simulink library "waveFlow_ul"  (R2018b)
settings: Solver=VariableStepAuto  StartTime=0.0  StopTime=10.0  RelTol=1e-3
undefined symbols (not defined in the file): e, initializeBussesFromBlock
settings Model: Creator=mcobb  LastModifiedBy=mcobb

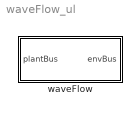
== system waveFlow_ul ==
  waveFlow : Subsystem  LoadFcn=initializeBussesFromBlock(gcb)  InitFcn=initializeBussesFromBlock(gcb)  StartFcn=initializeBussesFromBlock(gcb)  mask{e=e}
      mask prompts: e "Wave Flow Object"

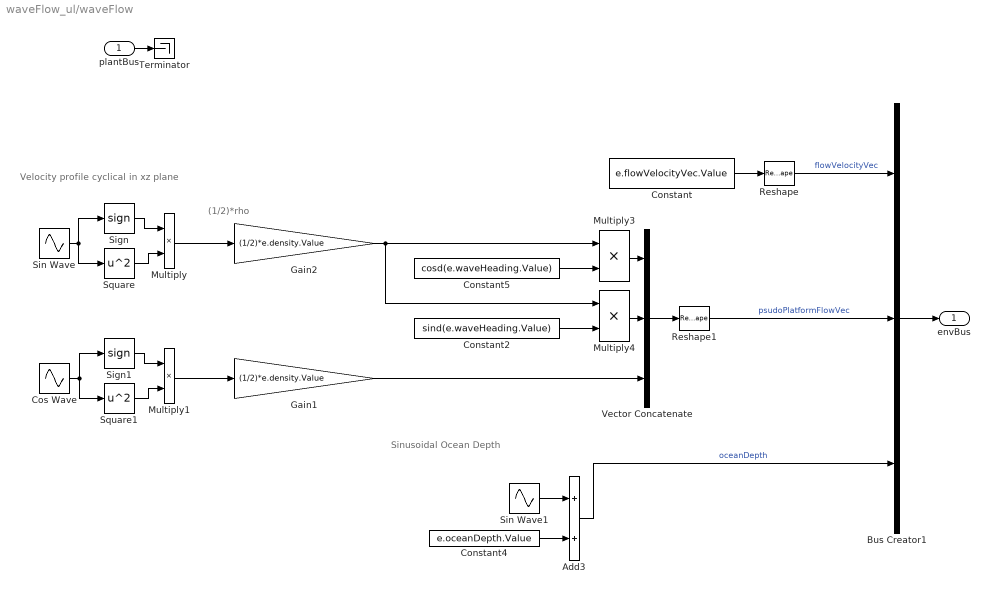
== system waveFlow_ul/waveFlow ==
  note: (1/2)*rho
  note: Velocity profile cyclical
      | in xz plane
  note: Sinusoidal Ocean Depth
  plantBus : Inport  OutDataTypeStr=Bus: plantBus
  Add3 : Sum
  Bus Creator1 : BusCreator  Inputs=3  OutDataTypeStr=Bus:envBus
  Constant : Constant  Value=e.flowVelocityVec.Value
  Constant2 : Constant  Value=sind(e.waveHeading.Value)
  Constant4 : Constant  Value=e.oceanDepth.Value
  Constant5 : Constant  Value=cosd(e.waveHeading.Value)
  Cos Wave : Sin  Amplitude=e.pltfrmAppFlwMag.Value  Frequency=2*pi/e.wavePeriod.Value  Phase=pi/2  SampleTime=0
  Gain1 : Gain  Gain=(1/2)*e.density.Value
  Gain2 : Gain  Gain=(1/2)*e.density.Value
  Multiply{,1,3..4} (4 alike) : Product
  Reshape : Reshape  OutputDimensionality=Column vector (2-D)
  Reshape1 : Reshape  OutputDimensionality=Column vector (2-D)
  Sign : Signum
  Sign1 : Signum
  Sin Wave : Sin  Amplitude=e.pltfrmAppFlwMag.Value  Frequency=2*pi/e.wavePeriod.Value  SampleTime=0
  Sin Wave1 : Sin  Amplitude=e.waveAmplitude.Value  Frequency=2*pi/e.wavePeriod.Value  SampleTime=0
  Square : Math  Operator=square  SaturateOnIntegerOverflow=on
  Square1 : Math  Operator=square  SaturateOnIntegerOverflow=on
  Terminator : Terminator
  Vector Concatenate : Concatenate  NumInputs=3
  envBus : Outport  OutDataTypeStr=Bus: envBus
  wires:
  Bus Creator1/1 -> envBus/1
  Constant/1 -> Reshape/1
  Reshape/1 -> Bus Creator1/1  "flowVelocityVec"
  Reshape1/1 -> Bus Creator1/2  "psudoPlatformFlowVec"
  Vector Concatenate/1 -> Reshape1/1
  Gain1/1 -> Vector Concatenate/3
  Gain2/1 -> Multiply3/1, Multiply4/1
  Sin Wave/1 -> Square/1, Sign/1
  Multiply/1 -> Gain2/1
  Square/1 -> Multiply/2
  Sign/1 -> Multiply/1
  Sign1/1 -> Multiply1/1
  Square1/1 -> Multiply1/2
  Multiply1/1 -> Gain1/1
  Cos Wave/1 -> Sign1/1, Square1/1
  Sin Wave1/1 -> Add3/1
  Add3/1 -> Bus Creator1/3  "oceanDepth"
  Constant4/1 -> Add3/2
  Multiply3/1 -> Vector Concatenate/1
  Constant2/1 -> Multiply4/2
  Multiply4/1 -> Vector Concatenate/2
  Constant5/1 -> Multiply3/2
  plantBus/1 -> Terminator/1
